simulink model "modelGreenHydrogenPlant"  (R2025a)
settings: Solver=ode1  StartTime=0.0  StopTime=exe.tsim  FixedStep=exe.tstep  RelTol=1e-3
undefined symbols (not defined in the file): Chosen_Strategy, DiscIntNeverNeededParam, ELY, ESS, exe, fb, Grid, grid, Ib2, Kc, kd, Ki_cc_cp, Ki_Inertia_Less, Kp_cc_cp, kp_GFo, Kp_Inertia_Less, PV, R, Rload, Sb, SCLR, t_ELY_on, Theta_Vvsc0, Time_Step, Va0, Vb0, Vb1, Vb2, Vc0, Vm0, VSC01_id0, Vvsc0, wb, Zb
libraries: spsSeriesRLCBranchLib x18, spsCurrentMeasurementLib x17, spsVoltageMeasurementLib x15, Control_Lib x13, spsRMSLib x8, simulink x8, spsabctodq0Lib x7, spsThreePhaseBreakerLib x5, spsPowerdq0InstantaneousLib x4, spsGroundLib x3, spsUniversalBridgeLib x3, spsControlledVoltageSourceLib x3
(part 3 of 3)

== system modelGreenHydrogenPlant/Supercapacitor/GFM_VC_newwith_Pvirt IDEAL_VSC/Control loops2/Power Control Loops1 ==
  P_mes : Inport
  P_set : Inport  Port=2
  delta_PLL : Inport  Port=3
  w_PLL : Inport  Port=4
  sat : Inport  Port=5
  Vg_rms : Inport  Port=6
  Compare To Constant : simulink/Logic and Bit Operations/Compare To Constant  relop===  const=1  OutDataTypeStr=boolean
  Compare To Constant1 : simulink/Logic and Bit Operations/Compare To Constant  relop===  const=2  OutDataTypeStr=boolean
  Compare To Constant2 : simulink/Logic and Bit Operations/Compare To Constant  relop===  const=3  OutDataTypeStr=boolean
  Inertia Less : Subsystem
  Multiport Switch : MultiPortSwitch  SaturateOnIntegerOverflow=off  InputSameDT=off
  Multiport Switch1 : MultiPortSwitch  SaturateOnIntegerOverflow=off  InputSameDT=off
  Mux : Mux  Inputs=[1 1]
  PI Controler : Subsystem
  Trigonometric Function : Trigonometry  Operator=cos
  Trigonometric Function1 : Trigonometry
  VSM : Subsystem
  w_set{1..4} (4 alike) : Constant  Value=Chosen_Strategy
  w_set_pu : Constant
  f : Outport  PortDimensions=1  VectorParamsAs1DForOutWhenUnconnected=off
  Theta : Outport  Port=2  VectorParamsAs1DForOutWhenUnconnected=off
  CosSinTheta : Outport  Port=3  PortDimensions=2  VectorParamsAs1DForOutWhenUnconnected=off
  wires:
  Trigonometric Function1/1 -> Mux/2
  Mux/1 -> CosSinTheta/1
  Trigonometric Function/1 -> Mux/1
  Compare To Constant2/1 -> PI Controler/Enable
  Compare To Constant1/1 -> VSM/Enable
  Compare To Constant/1 -> Inertia Less/Enable
  w_set4/1 -> Compare To Constant2/1
  w_set2/1 -> Compare To Constant1/1
  w_set3/1 -> Compare To Constant/1
  Inertia Less/1(frequency) -> Multiport Switch/2
  Multiport Switch/1 -> f/1
  Inertia Less/2(theta) -> Multiport Switch1/2
  VSM/2(theta) -> Multiport Switch1/3
  w_set1/1 -> Multiport Switch/1, Multiport Switch1/1
  VSM/1(frequency) -> Multiport Switch/3
  PI Controler/1(frequency) -> Multiport Switch/4
  PI Controler/2(theta) -> Multiport Switch1/4
  w_set_pu/1 -> PI Controler/3(w_set_pu)
  w_PLL/1 -> Inertia Less/4(w_PLL), VSM/3(w_PLL)
  delta_PLL/1 -> Inertia Less/3(delta_PLL)
  P_set/1 -> Inertia Less/2(P_set), VSM/2(P_set), PI Controler/2(P_set)
  P_mes/1 -> Inertia Less/1(P_mes), VSM/1(P_mes), PI Controler/1(P_mes)
  Multiport Switch1/1 -> Theta/1, Trigonometric Function1/1, Trigonometric Function/1
  sat/1 -> PI Controler/4(sat)
  Vg_rms/1 -> PI Controler/5(Vg_rms)

== system modelGreenHydrogenPlant/Supercapacitor/GFM_VC_newwith_Pvirt IDEAL_VSC/Control loops2/Transient Damping Resistance ==
  ig_dq : Inport
  Filter w_LF : Subsystem
      mask Display: disp('\omega_{LF} / (s + \omega_{LF})','texmode','on')
  Sum5 : Sum  Inputs=|+-
  nq1 : Gain  Gain=Rv
  "Delta_E_dq " : Outport  VectorParamsAs1DForOutWhenUnconnected=off
  wires:
  nq1/1 -> Filter w_LF/1(e), Sum5/2
  Filter w_LF/1(s) -> Sum5/1
  Sum5/1 -> "Delta_E_dq "/1
  ig_dq/1 -> nq1/1

== system modelGreenHydrogenPlant/Supercapacitor/GFM_VC_newwith_Pvirt IDEAL_VSC/Control loops2/Virtual Active Power calculation ==
  Voltage+ : Inport
  Current+ : Inport  Port=2
  Add2 : Sum
  Demux : Demux  Outputs=2
  Demux1 : Demux  Outputs=2
  Product : Product
  Product1 : Product
  Virtual Active Power : Outport
  wires:
  Product1/1 -> Add2/2
  Product/1 -> Add2/1
  Voltage+/1 -> Demux/1
  Current+/1 -> Demux1/1
  Demux/1 -> Product/2
  Demux/2 -> Product1/1
  Demux1/1 -> Product/1
  Demux1/2 -> Product1/2
  Add2/1 -> Virtual Active Power/1

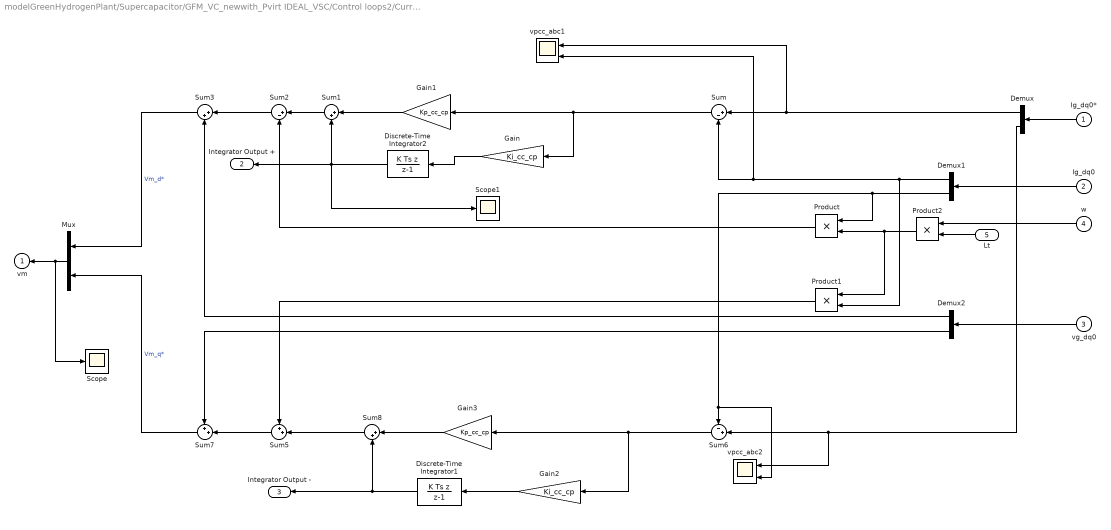
== system modelGreenHydrogenPlant/Supercapacitor/GFM_VC_newwith_Pvirt IDEAL_VSC/Control loops2/Current Limitation2/Current control ==
  Ig_dq0* : Inport
  Ig_dq0 : Inport  Port=2
  vg_dq0 : Inport  Port=3
  w : Inport  Port=4
  Lt : Inport  Port=5
  Demux : Demux  Outputs=2
  Demux1 : Demux  Outputs=2
  Demux2 : Demux  Outputs=2
  Discrete-Time Integrator1 : DiscreteIntegrator  IntegratorMethod=Integration: Backward Euler  SampleTime=Output_Delay  ICPrevOutput=DiscIntNeverNeededParam  ICPrevScaledInput=DiscIntNeverNeededParam
  Discrete-Time Integrator2 : DiscreteIntegrator  IntegratorMethod=Integration: Backward Euler  SampleTime=Output_Delay  ICPrevOutput=DiscIntNeverNeededParam  ICPrevScaledInput=DiscIntNeverNeededParam
  Gain : Gain  Gain=Ki_cc_cp
  Gain1 : Gain  Gain=Kp_cc_cp
  Gain2 : Gain  Gain=Ki_cc_cp
  Gain3 : Gain  Gain=Kp_cc_cp
  Mux : Mux  Inputs=2
  Product : Product  RndMeth=Zero
  Product1 : Product  RndMeth=Zero
  Product2 : Product  RndMeth=Zero
  Scope : Scope
      settings: ActiveDisplayYMinimum=-10.97849  ActiveDisplayYMaximum=3.98239
  Scope1 : Scope
      settings: ActiveDisplayYMinimum=-0.00069  ActiveDisplayYMaximum=0.00696
  Sum : Sum  Inputs=|+-
  Sum1 : Sum  Inputs=|++
  Sum2 : Sum  Inputs=|+-
  Sum3 : Sum  Inputs=|++
  Sum5 : Sum  Inputs=++|
  Sum6 : Sum  Inputs=-+|
  Sum7 : Sum  Inputs=++|
  Sum8 : Sum  Inputs=|++
  vpcc_abc1 : Scope  NumInputPorts=2
      settings: ActiveDisplayYMinimum=-0.30175  ActiveDisplayYMaximum=1.48559  DataLoggingVariableName=ScopeData2
  vpcc_abc2 : Scope  NumInputPorts=2
      settings: ActiveDisplayYMinimum=-1.30263  ActiveDisplayYMaximum=0.92364
  vm : Outport  InitialOutput=0  VectorParamsAs1DForOutWhenUnconnected=off
  Integrator Output + : Outport  Port=2
  Integrator Output - : Outport  Port=3
  wires:
  w/1 -> Product2/1
  Sum/1 -> Gain/1, Gain1/1
  Sum7/1 -> Mux/2  "Vm_q*"
  Sum3/1 -> Mux/1  "Vm_d*"
  Sum5/1 -> Sum7/2
  Product1/1 -> Sum5/1
  Demux/2 -> vpcc_abc2/1, Sum6/2
  Sum2/1 -> Sum3/1
  Product/1 -> Sum2/2
  Product2/1 -> Product1/1, Product/2
  Demux1/1 -> vpcc_abc1/2, Sum/2, Product1/2
  Ig_dq0/1 -> Demux1/1
  vg_dq0/1 -> Demux2/1
  Ig_dq0*/1 -> Demux/1
  Mux/1 -> Scope/1, vm/1
  Demux1/2 -> vpcc_abc2/2, Sum6/1, Product/1
  Demux2/1 -> Sum3/2
  Sum1/1 -> Sum2/1
  Sum8/1 -> Sum5/2
  Demux2/2 -> Sum7/1
  Gain/1 -> Discrete-Time Integrator2/1
  Gain1/1 -> Sum1/1
  Gain3/1 -> Sum8/1
  Gain2/1 -> Discrete-Time Integrator1/1
  Sum6/1 -> Gain2/1, Gain3/1
  Discrete-Time Integrator1/1 -> Sum8/2, Integrator Output -/1
  Lt/1 -> Product2/2
  Demux/1 -> vpcc_abc1/1, Sum/1
  Discrete-Time Integrator2/1 -> Integrator Output +/1, Scope1/1, Sum1/2

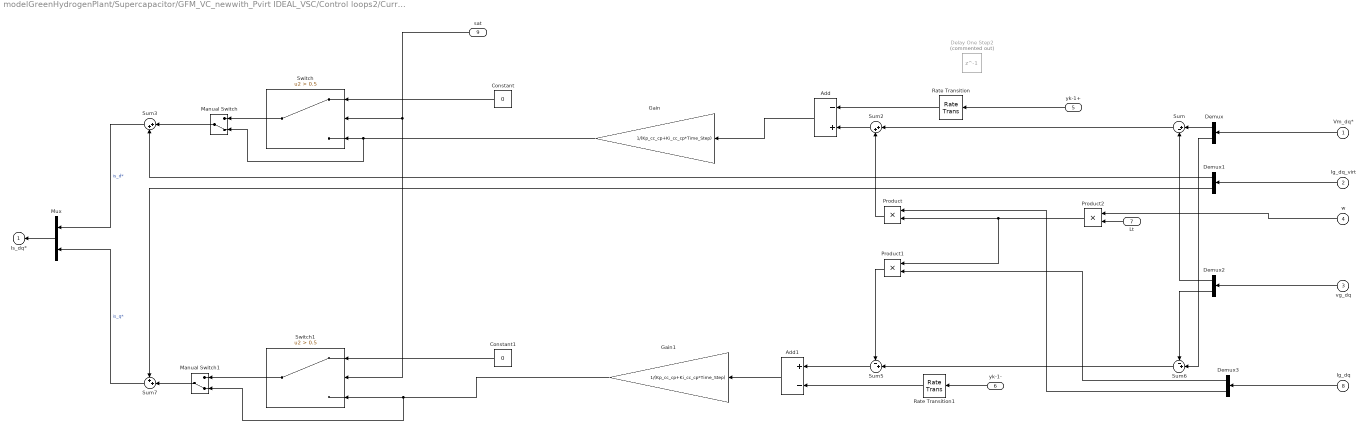
== system modelGreenHydrogenPlant/Supercapacitor/GFM_VC_newwith_Pvirt IDEAL_VSC/Control loops2/Current Limitation2/Inverse Current control ==
  Vm_dq* : Inport
  Ig_dq_virt : Inport  Port=2
  vg_dq : Inport  Port=3
  w : Inport  Port=4
  yk-1+ : Inport  Port=5
  yk-1- : Inport  Port=6
  Lt : Inport  Port=7
  Ig_dq : Inport  Port=8
  sat : Inport  Port=9
  Add : Sum  Inputs=-+
  Add1 : Sum  Inputs=+-
  Constant : Constant  Value=0
  Constant1 : Constant  Value=0
  Delay One Step2 : Delay  Commented=on  DelayLength=1  SampleTime=Time_Step
  Demux{,1..3} (4 alike) : Demux  Outputs=2
  Gain : Gain  Gain=1/(Kp_cc_cp+Ki_cc_cp*Time_Step)
  Gain1 : Gain  Gain=1/(Kp_cc_cp+Ki_cc_cp*Time_Step)
  Manual Switch : ManualSwitch  CurrentSetting=0
  Manual Switch1 : ManualSwitch  CurrentSetting=0
  Mux : Mux  Inputs=2
  Product : Product  RndMeth=Zero
  Product1 : Product  RndMeth=Zero
  Product2 : Product
  Rate Transition : RateTransition  OutPortSampleTime=Output_Delay
  Rate Transition1 : RateTransition  OutPortSampleTime=Output_Delay
  Sum : Sum  Inputs=|+-
  Sum2 : Sum  Inputs=|++
  Sum3 : Sum  Inputs=|++
  Sum5 : Sum  Inputs=-+|
  Sum6 : Sum  Inputs=-+|
  Sum7 : Sum  Inputs=++|
  Switch : Switch  Criteria=u2 > Threshold  Threshold=0.5  SaturateOnIntegerOverflow=off  InputSameDT=off
  Switch1 : Switch  Criteria=u2 > Threshold  Threshold=0.5  SaturateOnIntegerOverflow=off  InputSameDT=off
  Is_dq* : Outport  InitialOutput=0  VectorParamsAs1DForOutWhenUnconnected=off
  wires:
  Ig_dq_virt/1 -> Demux1/1
  Vm_dq*/1 -> Demux/1
  Demux/1 -> Sum/1
  Demux1/1 -> Sum3/2
  Sum/1 -> Sum2/1
  Product2/1 -> Product1/1, Product/2
  Sum2/1 -> Add/2
  Mux/1 -> Is_dq*/1
  Demux/2 -> Sum6/2
  Sum6/1 -> Sum5/2
  Sum3/1 -> Mux/1  "is_d*"
  Sum7/1 -> Mux/2  "is_q*"
  w/1 -> Product2/1
  Demux1/2 -> Sum7/1
  yk-1+/1 -> Rate Transition/1
  Rate Transition/1 -> Add/1
  Add/1 -> Gain/1
  Add1/1 -> Gain1/1
  Sum5/1 -> Add1/1
  yk-1-/1 -> Rate Transition1/1
  Rate Transition1/1 -> Add1/2
  Product1/1 -> Sum5/1
  Product/1 -> Sum2/2
  vg_dq/1 -> Demux2/1
  Demux2/2 -> Sum6/1
  Demux2/1 -> Sum/2
  Lt/1 -> Product2/2
  Ig_dq/1 -> Demux3/1
  Demux3/2 -> Product/1
  Demux3/1 -> Product1/2
  sat/1 -> Switch1/2, Switch/2
  Gain/1 -> Manual Switch/2, Switch/3
  Constant/1 -> Switch/1
  Constant1/1 -> Switch1/1
  Gain1/1 -> Manual Switch1/2, Switch1/3
  Manual Switch/1 -> Sum3/1
  Switch/1 -> Manual Switch/1
  Manual Switch1/1 -> Sum7/2
  Switch1/1 -> Manual Switch1/1

== system modelGreenHydrogenPlant/Supercapacitor/GFM_VC_newwith_Pvirt IDEAL_VSC/Control loops2/Current reference generation/RMS2 ==
  Is_dq* : Inport
  Demux : Demux  Outputs=2
  Sqrt : Sqrt
  Square : Math  Operator=square
  Square1 : Math  Operator=square
  Sum : Sum  Inputs=|++
  Out1 : Outport
  wires:
  Demux/2 -> Square1/1
  Is_dq*/1 -> Demux/1
  Demux/1 -> Square/1
  Sqrt/1 -> Out1/1
  Square1/1 -> Sum/2
  Square/1 -> Sum/1
  Sum/1 -> Sqrt/1

== system modelGreenHydrogenPlant/Supercapacitor/GFM_VC_newwith_Pvirt IDEAL_VSC/Control loops2/Current reference generation/Subsystem ==
  In1 : Inport
  tau_f : Inport  Port=2
  Integrator : Integrator  InitialConditionSource=external  InitialCondition=1
  Product : Product  Inputs=/*
  Sum2 : Sum  Inputs=|+-
  Out1 : Outport
  wires:
  Product/1 -> Integrator/1
  Sum2/1 -> Product/2
  Integrator/1 -> Sum2/2, Out1/1
  tau_f/1 -> Product/1
  In1/1 -> Integrator/2, Sum2/1

== system modelGreenHydrogenPlant/Supercapacitor/GFM_VC_newwith_Pvirt IDEAL_VSC/Control loops2/Current reference generation/Subsystem1 ==
  tau_f : Inport
  In1 : Inport  Port=2
  Integrator : Integrator  InitialConditionSource=external
  Product : Product  Inputs=/*
  Sum2 : Sum  Inputs=|+-
  Out1 : Outport
  wires:
  Product/1 -> Integrator/1
  Sum2/1 -> Product/2
  Integrator/1 -> Sum2/2, Out1/1
  In1/1 -> Sum2/1, Integrator/2
  tau_f/1 -> Product/1

== system modelGreenHydrogenPlant/Supercapacitor/GFM_VC_newwith_Pvirt IDEAL_VSC/Control loops2/Power Control Loops1/Inertia Less ==
  P_mes : Inport
  P_set : Inport  Port=2
  delta_PLL : Inport  Port=3
  w_PLL : Inport  Port=4
  Enable : EnablePort
  2*pi : Constant  Value=2*pi
  2*pi1 : Constant
  2*pi3 : Constant  Value=Val_Freq_Support
  2*pi4 : Constant  Value=0
  Gain : Gain  Commented=on  Gain=Kp_Inertia_Less
  Gain1 : Gain  Gain=Kp_Inertia_Less
  Integrator : Integrator  Commented=on  InitialConditionSource=external
  Integrator2 : Integrator  InitialCondition=(Theta0_VSC)*pi/180-Theta0*pi/180
  Math Function : Math  Operator=mod  SignedPower=on
  Sum : Sum  Inputs=++-
  Sum1 : Sum  Inputs=++|
  Sum2 : Sum  Inputs=|+-
  Sum5 : Sum  Inputs=++|
  Sum6 : Sum  Inputs=|+-
  Sum7 : Sum  Inputs=++|
  Switch : Switch  Criteria=u2 > Threshold  Threshold=0.5  SaturateOnIntegerOverflow=off  InputSameDT=off
  mp : Gain  Commented=on  Gain=Ki_Inertia_Less
  mp2 : Gain  Gain=1/R
  mp3 : Gain  Gain=wb
  frequency : Outport  VectorParamsAs1DForOutWhenUnconnected=off
  theta : Outport  Port=2  VectorParamsAs1DForOutWhenUnconnected=off
  wires:
  Sum5/1 -> frequency/1
  Switch/1 -> Sum7/2
  Gain1/1 -> Sum/1
  Gain/1 -> Integrator/2, Sum/3
  Integrator/1 -> Sum/2
  2*pi4/1 -> Switch/3
  2*pi3/1 -> Switch/2
  mp2/1 -> Switch/1
  Integrator2/1 -> Sum1/2
  w_PLL/1 -> Sum5/2, Sum6/2
  delta_PLL/1 -> Sum1/1  "delta_m_ref"
  mp/1 -> Integrator/1
  mp3/1 -> Integrator2/1
  Sum/1 -> mp3/1, Sum5/1  "delta_w"
  Math Function/1 -> theta/1
  P_mes/1 -> Sum2/2, Gain/1
  Sum7/1 -> Sum2/1  "P_ref"
  P_set/1 -> Sum7/1
  Sum6/1 -> mp2/1
  2*pi1/1 -> Sum6/1
  2*pi/1 -> Math Function/2
  Sum1/1 -> Math Function/1  "delta_m_ref"
  Sum2/1 -> mp/1, Gain1/1

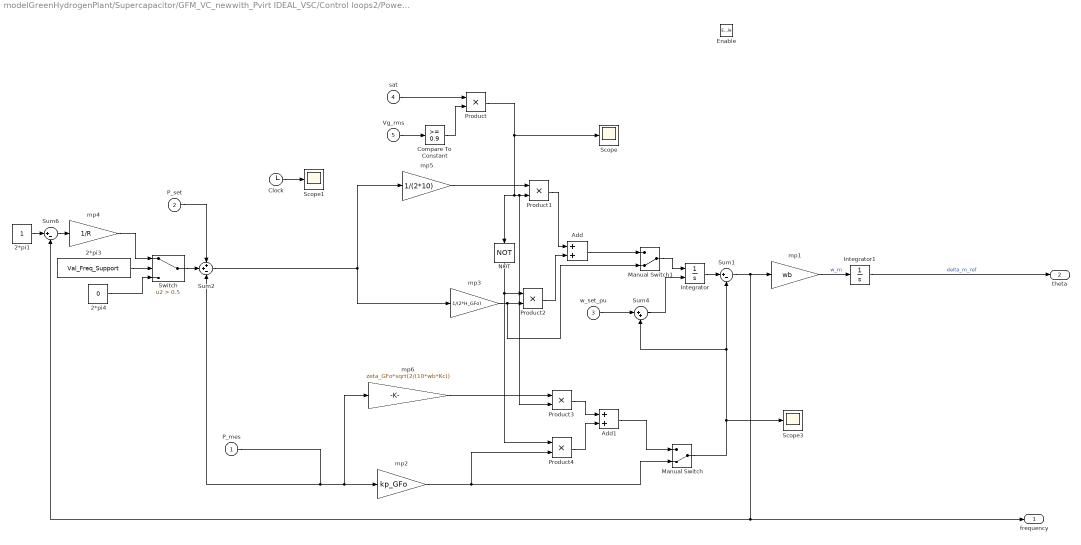
== system modelGreenHydrogenPlant/Supercapacitor/GFM_VC_newwith_Pvirt IDEAL_VSC/Control loops2/Power Control Loops1/PI Controler ==
  P_mes : Inport
  P_set : Inport  Port=2
  w_set_pu : Inport  Port=3
  sat : Inport  Port=4
  Vg_rms : Inport  Port=5
  Enable : EnablePort
  2*pi1 : Constant
  2*pi3 : Constant  Value=Val_Freq_Support
  2*pi4 : Constant  Value=0
  Add : Sum
  Add1 : Sum
  Clock : Clock
  Compare To Constant : simulink/Logic and Bit Operations/Compare To Constant  relop=>=  const=0.9  OutDataTypeStr=boolean
  Integrator : Integrator  InitialConditionSource=external
  Integrator1 : Integrator  InitialCondition=(Theta0_VSC)*pi/180
  Manual Switch : ManualSwitch  CurrentSetting=0
  Manual Switch1 : ManualSwitch  CurrentSetting=0
  NOT : Logic  Operator=NOT  IconShape=distinctive  AllPortsSameDT=off  OutDataTypeStr=boolean
  Product{,1..4} (5 alike) : Product
  Scope : Scope
      settings: ActiveDisplayYMinimum=-0.125  ActiveDisplayYMaximum=1.125  DataLoggingVariableName=ScopeData2
  Scope1 : Scope
      settings: ActiveDisplayYMinimum=-0.25  ActiveDisplayYMaximum=2.25
  Scope3 : Scope
      settings: ActiveDisplayYMinimum=0.01909  ActiveDisplayYMaximum=0.01939  DataLoggingVariableName=ScopeData3
  Sum1 : Sum  Inputs=|+-
  Sum2 : Sum  Inputs=++-
  Sum4 : Sum  Inputs=|++
  Sum6 : Sum  Inputs=|+-
  Switch : Switch  Criteria=u2 > Threshold  Threshold=0.5  SaturateOnIntegerOverflow=off  InputSameDT=off
  mp1 : Gain  Gain=wb
  mp2 : Gain  Gain=kp_GFo
  mp3 : Gain  Gain=1/(2*H_GFo)
  mp4 : Gain  Gain=1/R
  mp5 : Gain  Gain=1/(2*10)
  mp6 : Gain  Gain=zeta_GFo*sqrt(2/(10*wb*Kc))
  frequency : Outport  VectorParamsAs1DForOutWhenUnconnected=off
  theta : Outport  Port=2  VectorParamsAs1DForOutWhenUnconnected=off
  wires:
  Switch/1 -> Sum2/2
  2*pi4/1 -> Switch/3
  Sum6/1 -> mp4/1
  2*pi3/1 -> Switch/2
  2*pi1/1 -> Sum6/1
  mp4/1 -> Switch/1
  Sum4/1 -> Integrator/2
  P_mes/1 -> Sum2/3, mp6/1, mp2/1
  mp1/1 -> Integrator1/1  "w_m"
  Sum1/1 -> Sum6/2, frequency/1, mp1/1
  Integrator/1 -> Sum1/1
  P_set/1 -> Sum2/1
  w_set_pu/1 -> Sum4/1
  Integrator1/1 -> theta/1  "delta_m_ref"
  Sum2/1 -> mp3/1, mp5/1
  Vg_rms/1 -> Compare To Constant/1
  sat/1 -> Product/1
  Compare To Constant/1 -> Product/2
  mp6/1 -> Product3/1
  mp2/1 -> Product4/2, Manual Switch/2
  Clock/1 -> Scope1/1
  Add1/1 -> Manual Switch/1
  Manual Switch/1 -> Scope3/1, Sum1/2, Sum4/2
  Manual Switch1/1 -> Integrator/1
  mp5/1 -> Product1/1
  Product/1 -> Scope/1, Product3/2, Product1/2, NOT/1
  Product1/1 -> Add/1
  NOT/1 -> Product4/1, Product2/1
  Product2/1 -> Add/2
  Add/1 -> Manual Switch1/1
  mp3/1 -> Manual Switch1/2, Product2/2
  Product3/1 -> Add1/1
  Product4/1 -> Add1/2

== system modelGreenHydrogenPlant/Supercapacitor/GFM_VC_newwith_Pvirt IDEAL_VSC/Control loops2/Power Control Loops1/VSM ==
  P_mes : Inport
  P_set : Inport  Port=2
  w_PLL : Inport  Port=3
  Enable : EnablePort
  2*pi1 : Constant
  2*pi3 : Constant  Value=Val_Freq_Support
  2*pi4 : Constant  Value=0
  Gain : Gain  Gain=kd
  Gain1 : Gain  Gain=1/(2*H_GFo)
  Integrator : Integrator  InitialCondition=1
  Integrator1 : Integrator  InitialCondition=Theta0_VSC*pi/180
  Sum : Sum  Inputs=|+-
  Sum1 : Sum  Inputs=++-
  Sum6 : Sum  Inputs=|+-
  Sum7 : Sum  Inputs=++|
  Switch : Switch  Criteria=u2 > Threshold  Threshold=0.5  SaturateOnIntegerOverflow=off  InputSameDT=off
  mp1 : Gain  Gain=1/R
  mp2 : Gain  Gain=wb
  frequency : Outport  VectorParamsAs1DForOutWhenUnconnected=off
  theta : Outport  Port=2  VectorParamsAs1DForOutWhenUnconnected=off
  wires:
  Gain1/1 -> Integrator/1
  Sum7/1 -> Sum1/2  "P_ref"
  Sum1/1 -> Gain1/1
  Gain/1 -> Sum1/1
  Sum/1 -> Gain/1
  w_PLL/1 -> Sum/1
  2*pi4/1 -> Switch/3
  2*pi3/1 -> Switch/2
  mp1/1 -> Switch/1
  2*pi1/1 -> Sum6/1
  Sum6/1 -> mp1/1
  P_set/1 -> Sum7/1
  Switch/1 -> Sum7/2
  mp2/1 -> Integrator1/1
  P_mes/1 -> Sum1/3
  Integrator/1 -> Sum6/2, frequency/1, mp2/1, Sum/2  "wm"
  Integrator1/1 -> theta/1  "delta_m_ref"

== system modelGreenHydrogenPlant/Supercapacitor/GFM_VC_newwith_Pvirt IDEAL_VSC/Control loops2/Transient Damping Resistance/Filter w_LF ==
  e : Inport
  1/T_LP : Gain  Gain=W_TVR  SaturateOnIntegerOverflow=on  OutDataTypeStr=Inherit: Same as input  ParamDataTypeStr=Inherit: Same as input
  Integrator : Integrator  InitialConditionSource=external  InitialCondition=[VSC01_id0*0.04]
  Sum1 : Sum  Inputs=|+-  InputSameDT=on  SaturateOnIntegerOverflow=on  OutDataTypeStr=Inherit: Same as first input
  s : Outport  VectorParamsAs1DForOutWhenUnconnected=off
  wires:
  e/1 -> Sum1/1, Integrator/2
  Integrator/1 -> s/1, Sum1/2
  1/T_LP/1 -> Integrator/1
  Sum1/1 -> 1/T_LP/1
